simulink model "Part4_1_2"  (R2022a)
settings: Solver=VariableStepAuto  StartTime=0.0  StopTime=200  RelTol=1e-3
undefined symbols (not defined in the file or in its folder): quant
settings Model: Creator=theod  LastModifiedBy=theod
settings DebuggingCC: UnconnectedInputMsg=warning  UnconnectedOutputMsg=warning  UnconnectedLineMsg=warning
settings RTWCC: DLArmComputeVersion=19.05

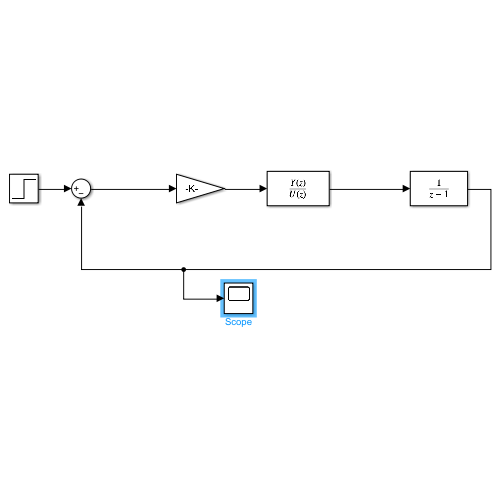
[thumbnail: Simulink's stored preview of the top-level diagram]
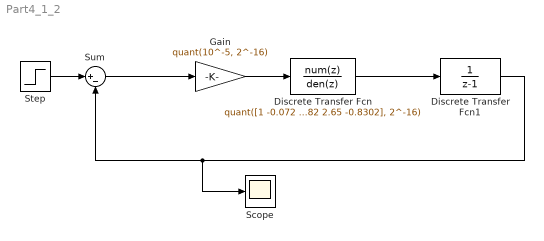
== system Part4_1_2 ==
  Discrete Transfer Fcn : DiscreteTransferFcn  Numerator=quant([1 -0.072 -0.2349], 2^-16)  Denominator="quant([1  -2.82 2.65 -0.8302], 2^-16)"  SampleTime=0.1
  Discrete Transfer Fcn1 : DiscreteTransferFcn  Denominator=[1 -1]  SampleTime=0.1
  Gain : Gain  Gain=quant(10^-5, 2^-16)
  Scope : Scope
  Step : Step  SampleTime=0.1  VectorParams1D=off  ZeroCross=off
  Sum : Sum  Inputs=|+-
  wires:
  Discrete Transfer Fcn1/1 -> Scope/1, Sum/2
  Step/1 -> Sum/1
  Sum/1 -> Gain/1
  Gain/1 -> Discrete Transfer Fcn/1
  Discrete Transfer Fcn/1 -> Discrete Transfer Fcn1/1
